simulink model "Controller"  (R2016b)
settings: configuration reference "WheelSimConfiguration2016" (kept outside this file)
undefined symbols (not defined in the file): simulator
libraries: simulink_extras x2, simulink x1
settings Model: Creator=At  LastModifiedBy=At
settings ConfigSetRef: SourceLocation=Base Workspace

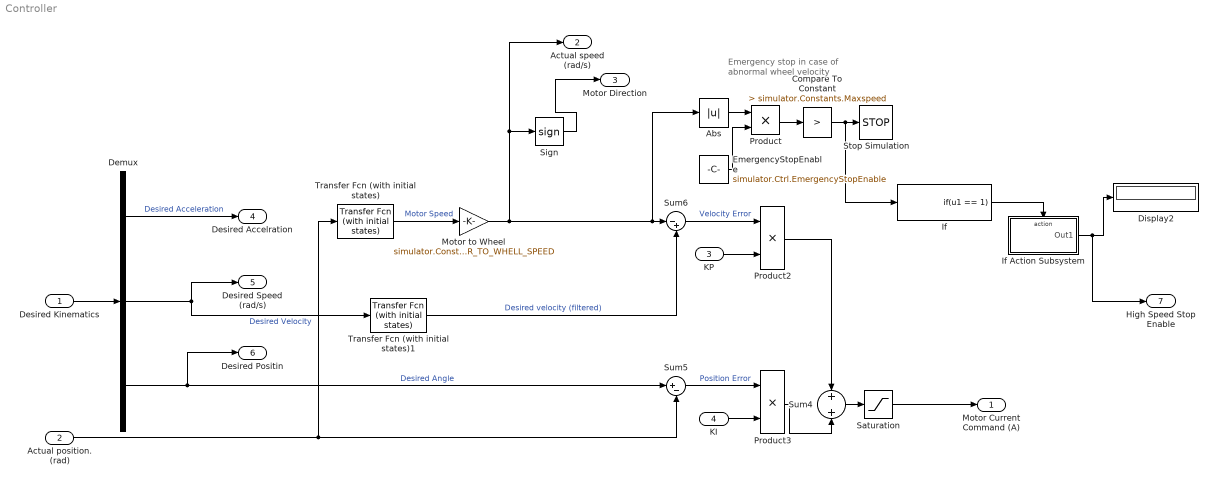
== system Controller ==
  note: Emergency stop in case of
      | abnormal wheel velocity
  Desired Kinematics : Inport
  Actual position. (rad) : Inport  Port=2
  KP : Inport  Port=3
  KI : Inport  Port=4
  Abs : Abs
  Compare To Constant : simulink/Logic and Bit Operations/Compare To Constant  relop=>  const=simulator.Constants.Maxspeed  OutDataTypeStr=boolean
  Demux : Demux  Outputs=3
  Display2 : Display
  EmergencyStopEnable : Constant  Value=simulator.Ctrl.EmergencyStopEnable
  If : If  IfExpression=u1 == 1  ShowElse=off
  If Action Subsystem : Subsystem  TreatAsAtomicUnit=on
  Motor to Wheel : Gain  Gain=simulator.Constants.MOTOR_TO_WHELL_SPEED
  Product : Product  RndMeth=Zero
  Product2 : Product  RndMeth=Zero
  Product3 : Product  RndMeth=Zero
  Saturation : Saturate  UpperLimit=5  LowerLimit=-5
  Sign : Signum
  Stop Simulation : Stop
  Sum4 : Sum
  Sum5 : Sum  Inputs=|+-
  Sum6 : Sum  Inputs=|-+
  Transfer Fcn (with initial states) : simulink_extras/Additional Linear/Transfer Fcn (with initial states)  N=[1 0]  D="[1  0.5]"  X0=0
  Transfer Fcn (with initial states)1 : simulink_extras/Additional Linear/Transfer Fcn (with initial states)  N=[1]  D="[1  0.5]"  X0=0
  Motor Current Command (A) : Outport
  Actual speed (rad/s) : Outport  Port=2
  Motor Direction : Outport  Port=3
  Desired Accelration : Outport  Port=4
  Desired Speed (rad/s) : Outport  Port=5
  Desired Positin : Outport  Port=6
  High Speed Stop Enable : Outport  Port=7
  wires:
  Actual position. (rad)/1 -> Transfer Fcn (with initial states)/1, Sum5/2
  Transfer Fcn (with initial states)1/1 -> Sum6/2  "Desired velocity (filtered)"
  Desired Kinematics/1 -> Demux/1
  Demux/2 -> Transfer Fcn (with initial states)1/1, Desired Speed (rad/s)/1  "Desired Velocity"
  Demux/3 -> Desired Positin/1, Sum5/1  "Desired Angle"
  Demux/1 -> Desired Accelration/1  "Desired Acceleration"
  Compare To Constant/1 -> If/1, Stop Simulation/1
  KI/1 -> Product3/2
  KP/1 -> Product2/2
  Sum5/1 -> Product3/1  "Position Error"
  Sum6/1 -> Product2/1  "Velocity Error"
  Sum4/1 -> Saturation/1
  Saturation/1 -> Motor Current Command (A)/1
  Abs/1 -> Product/1
  Product/1 -> Compare To Constant/1
  EmergencyStopEnable/1 -> Product/2
  Product2/1 -> Sum4/1
  Product3/1 -> Sum4/2
  Transfer Fcn (with initial states)/1 -> Motor to Wheel/1  "Motor Speed"
  Sign/1 -> Motor Direction/1
  Motor to Wheel/1 -> Sum6/1, Abs/1, Sign/1, Actual speed (rad/s)/1
  If/1 -> If Action Subsystem/Action
  If Action Subsystem/1(Out1) -> High Speed Stop Enable/1, Display2/1

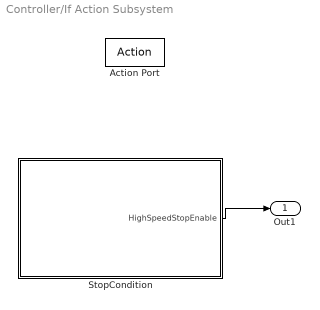
== system Controller/If Action Subsystem ==
  Action Port : ActionPort  ActionType=then
  StopCondition : MATLAB Function  TreatAsAtomicUnit=on
  Out1 : Outport
  wires:
  StopCondition/1(HighSpeedStopEnable) -> Out1/1

== matlab function Controller/If Action Subsystem/StopCondition ==
  data: HighSpeedStopEnable output
function HighSpeedStopEnable   = stopcondition(  )

%% This function determines the reason for stoping the system


    
HighSpeedStopEnable=1;
